simulink model "sim_process_power"  (R2021a)
settings: Solver=VariableStepAuto  StartTime=0.0  StopTime=0.1  MaxStep=1/25e3  RelTol=1e-3
undefined symbols (not defined in the file): meas4
libraries: spsAlphaBetaZerotodq0Lib x2, spsabctoAlphaBetaZeroLib x2, spsPLL3phLib x1, spsPower3phInstantaneousLib x1, eePowerMeasurement x1, spsRMSLib x1, eeSinusoidalMeasurementV2 x1, eeTransforms x1, spsTHDLib x1, eeTotalHarmonicDistorsion x1
settings Model: Creator=VMORAIS  LastModifiedBy=VMORAIS

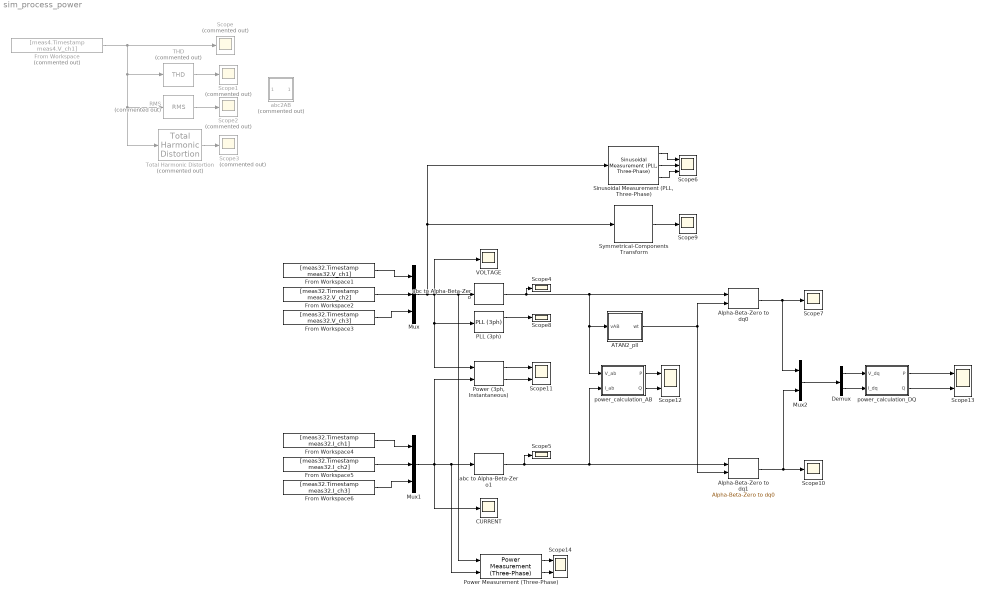
== system sim_process_power ==
  ATAN2_pll : Subsystem
  Alpha-Beta-Zero to dq0 : spsAlphaBetaZerotodq0Lib/Alpha-Beta-Zero to dq0  Alignment=90 degrees behind phase A axis
      settings: SourceProductBaseCode=PS
  Alpha-Beta-Zero to dq1 : spsAlphaBetaZerotodq0Lib/Alpha-Beta-Zero to dq0  Alignment=90 degrees behind phase A axis
      settings: SourceProductBaseCode=PS
  CURRENT : Scope
  Demux : Demux  Outputs=2
  From Workspace : FromWorkspace  Commented=on  VariableName=[meas4.Timestamp meas4.V_ch1]  SampleTime=meas4.Timestamp(2)-meas4.Timestamp(1)
  From Workspace1 : FromWorkspace  VariableName=[meas32.Timestamp meas32.V_ch1]  SampleTime=-1
  From Workspace2 : FromWorkspace  VariableName=[meas32.Timestamp meas32.V_ch2]  SampleTime=-1
  From Workspace3 : FromWorkspace  VariableName=[meas32.Timestamp meas32.V_ch3]  SampleTime=-1
  From Workspace4 : FromWorkspace  VariableName=[meas32.Timestamp meas32.I_ch1]  SampleTime=-1
  From Workspace5 : FromWorkspace  VariableName=[meas32.Timestamp meas32.I_ch2]  SampleTime=-1
  From Workspace6 : FromWorkspace  VariableName=[meas32.Timestamp meas32.I_ch3]  SampleTime=-1
  Mux : Mux  Inputs=3
  Mux1 : Mux  Inputs=3
  Mux2 : Mux  Inputs=2
  PLL (3ph) : spsPLL3phLib/PLL (3ph)  Fmin=59  Par_Init=[0, 60]  ParK=[18, 3200, 1]  TcD=1e-4  MaxRateChangeFreq=120  FilterCutOffFreq=100  Ts=0  AGC=on
  "Power (3ph, Instantaneous)" : spsPower3phInstantaneousLib/Power (3ph, Instantaneous)
  Power Measurement (Three-Phase) : eePowerMeasurement/Power Measurement (Three-Phase)  LabelModeActiveChoice=Continuous  F=60  K=[0 1 2 3]  Seq=Positive  Ts=0
      settings: SourceProductBaseCode=PS
  RMS : spsRMSLib/RMS  Commented=on  TrueRMS=on  Freq=50  RMSInit=230  Ts=0
  Scope{,1..3} (4 alike) : Scope  Commented=on
  Scope{4..5,7..10} (6 alike) : Scope
  Scope{11..14} (4 alike) : Scope  NumInputPorts=2
  Scope6 : Scope  NumInputPorts=3
  "Sinusoidal Measurement (PLL, Three-Phase)" : eeSinusoidalMeasurementV2/Sinusoidal Measurement (PLL, Three-Phase)  Kp_LF=200  Ki_LF=2000  F0=60  Theta0=0  Ts=-1
      settings: SourceProductBaseCode=PS
  Symmetrical-Components Transform : eeTransforms/Symmetrical-Components Transform  PowerInvariant=off
      settings: SourceProductBaseCode=PS
  THD : spsTHDLib/THD  Commented=on  Freq=50  Ts=0
      settings: SourceProductBaseCode=PS
  Total Harmonic Distortion : eeTotalHarmonicDistorsion/Total Harmonic Distortion  Commented=on  f=50  Ts=-1
      settings: SourceProductBaseCode=PS
  VOLTAGE : Scope
  abc to Alpha-Beta-Zero : spsabctoAlphaBetaZeroLib/abc to Alpha-Beta-Zero
      settings: SourceProductBaseCode=PS
  abc to Alpha-Beta-Zero1 : spsabctoAlphaBetaZeroLib/abc to Alpha-Beta-Zero
      settings: SourceProductBaseCode=PS
  abc2AB : Subsystem  Commented=on
  power_calculation_AB : MATLAB Function  TreatAsAtomicUnit=on
  power_calculation_DQ : MATLAB Function  TreatAsAtomicUnit=on
  wires:
  From Workspace/1 -> Scope/1, THD/1, RMS/1, Total Harmonic Distortion/1
  THD/1 -> Scope1/1
  RMS/1 -> Scope2/1
  Total Harmonic Distortion/1 -> Scope3/1
  From Workspace2/1 -> Mux/2
  From Workspace1/1 -> Mux/1
  From Workspace3/1 -> Mux/3
  Mux/1 -> "Sinusoidal Measurement (PLL, Three-Phase)"/1, Symmetrical-Components Transform/1, Power Measurement (Three-Phase)/1, abc to Alpha-Beta-Zero/1, "Power (3ph, Instantaneous)"/1, PLL (3ph)/1, VOLTAGE/1
  PLL (3ph)/1 -> Scope8/1
  From Workspace6/1 -> Mux1/3
  From Workspace4/1 -> Mux1/1
  From Workspace5/1 -> Mux1/2
  Mux1/1 -> Power Measurement (Three-Phase)/2, abc to Alpha-Beta-Zero1/1, "Power (3ph, Instantaneous)"/2, CURRENT/1
  abc to Alpha-Beta-Zero1/1 -> Scope5/1, Alpha-Beta-Zero to dq1/1, power_calculation_AB/2(I_ab)
  "Power (3ph, Instantaneous)"/1 -> Scope11/1
  "Power (3ph, Instantaneous)"/2 -> Scope11/2
  power_calculation_AB/2(Q) -> Scope12/2
  power_calculation_AB/1(P) -> Scope12/1
  Alpha-Beta-Zero to dq1/1 -> Scope10/1, Mux2/2
  Alpha-Beta-Zero to dq0/1 -> Mux2/1, Scope7/1
  power_calculation_DQ/1(P) -> Scope13/1
  power_calculation_DQ/2(Q) -> Scope13/2
  Demux/1 -> power_calculation_DQ/1(V_dq)
  Demux/2 -> power_calculation_DQ/2(I_dq)
  Mux2/1 -> Demux/1
  abc to Alpha-Beta-Zero/1 -> Scope4/1, ATAN2_pll/1(vAB), power_calculation_AB/1(V_ab), Alpha-Beta-Zero to dq0/1
  ATAN2_pll/1(wt) -> Alpha-Beta-Zero to dq0/2, Alpha-Beta-Zero to dq1/2
  Symmetrical-Components Transform/1 -> Scope9/1
  Power Measurement (Three-Phase)/1 -> Scope14/1
  Power Measurement (Three-Phase)/2 -> Scope14/2
  "Sinusoidal Measurement (PLL, Three-Phase)"/1 -> Scope6/1
  "Sinusoidal Measurement (PLL, Three-Phase)"/2 -> Scope6/2
  "Sinusoidal Measurement (PLL, Three-Phase)"/3 -> Scope6/3

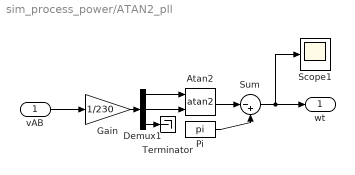
== system sim_process_power/ATAN2_pll ==
  vAB : Inport
  Atan2 : Trigonometry  Operator=atan2
  Demux1 : Demux  Outputs=3
  Gain : Gain  Gain=1/230
  Pi : Constant  Value=pi  OutDataTypeStr=Inherit: Inherit via back propagation
  Scope1 : Scope
  Sum : Sum  Inputs=|-+
  Terminator : Terminator
  wt : Outport
  wires:
  Atan2/1 -> Sum/1
  Demux1/2 -> Atan2/2
  Sum/1 -> Scope1/1, wt/1
  Demux1/1 -> Atan2/1
  Pi/1 -> Sum/2
  Gain/1 -> Demux1/1
  Demux1/3 -> Terminator/1
  vAB/1 -> Gain/1

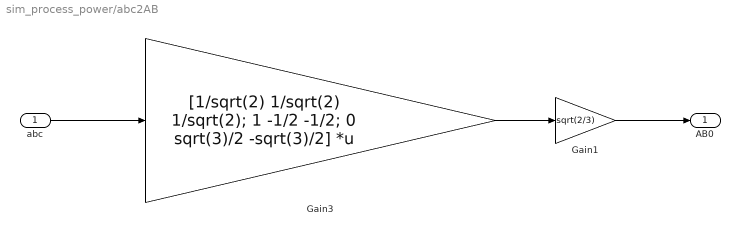
== system sim_process_power/abc2AB ==
  abc : Inport
  Gain1 : Gain  Gain=sqrt(2/3)  SaturateOnIntegerOverflow=on  OutDataTypeStr=Inherit: Same as input  ParamDataTypeStr=Inherit: Same as input
  Gain3 : Gain  Gain=[1/sqrt(2) 1/sqrt(2) 1/sqrt(2); 1 -1/2 -1/2; 0 sqrt(3)/2 -sqrt(3)/2]  Multiplication=Matrix(K*u) (u vector)  SaturateOnIntegerOverflow=on  OutDataTypeStr=Inherit: Same as input  ParamDataTypeStr=Inherit: Same as input
  AB0 : Outport
  wires:
  Gain1/1 -> AB0/1
  Gain3/1 -> Gain1/1
  abc/1 -> Gain3/1

== matlab function sim_process_power/power_calculation_AB ==
  data: V_ab input; P output; I_ab input; Q output
function [P,Q] = fcn(V_ab, I_ab)

%%ref: http://repositorium.sdum.uminho.pt/bitstream/1822/1864/1/ISIE-03_JLA.pdf
P = V_ab(1)*I_ab(1) + V_ab(2)*I_ab(2);
Q = V_ab(2)*I_ab(1) - V_ab(1)*I_ab(2);

== matlab function sim_process_power/power_calculation_DQ ==
  data: V_dq input; P output; I_dq input; Q output
function [P,Q] = fcn(V_dq, I_dq)

%%ref: http://repositorium.sdum.uminho.pt/bitstream/1822/1864/1/ISIE-03_JLA.pdf
P = 3/2 * V_dq(1) * I_dq(1);
Q = 3/2 * V_dq(1) * I_dq(2);
